simulink subsystem "WP_Guidance"  (R2021b)
settings: Solver=VariableStepAuto  StartTime=0.0  StopTime=10.0  RelTol=1e-3
undefined symbols (not defined in the file): ap, Earth, WGS84
libraries: mbdriLib x8, aerolibtransform2 x2
settings Model: Creator=promero  LastModifiedBy=promero

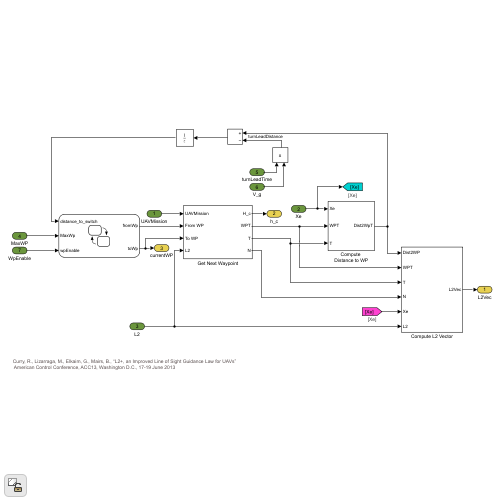
[thumbnail: Simulink's stored preview of the top-level diagram]
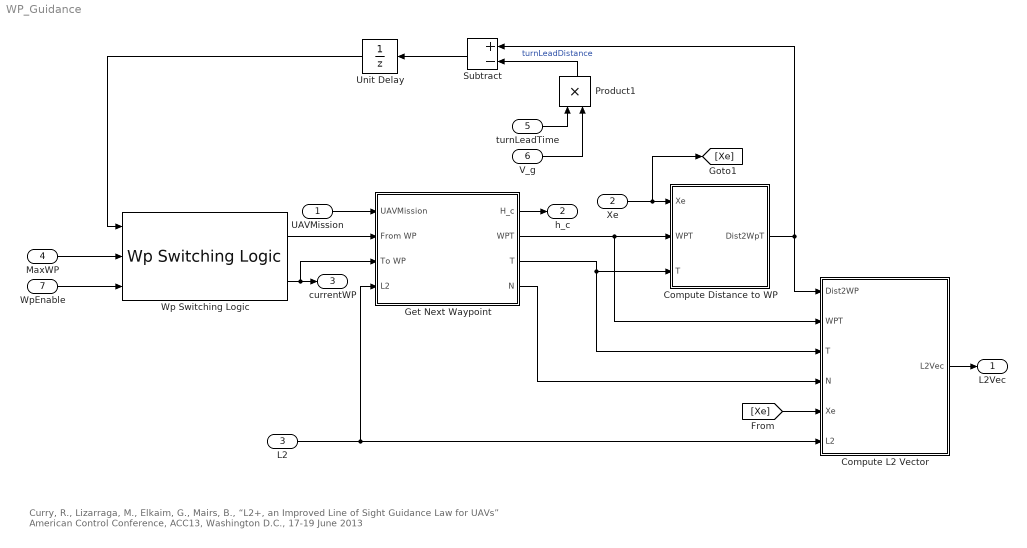
== system WP_Guidance ==
  note: Curry, R., Lizarraga, M., Elkaim, G., Mairs, B., “L2+, an Improved Line of Sight Guidance Law for UAVs”
      | American Control Conference, ACC13, Washington D.C., 17-19 June 2013
  UAVMission : Inport  RequirementInfo={} %GIDa_ee9cd0ca_ee46_4171_b2ca_c1436fe27e01
  Xe : Inport  RequirementInfo={} %GIDa_72129976_cf07_4668_8a2e_61079a25596c  Port=2
  L2 : Inport  RequirementInfo={} %GIDa_3bb9d2b1_49b6_4fd1_b19e_adcb7eb29e87  Port=3
  MaxWP : Inport  RequirementInfo={} %GIDa_a09e5540_0b09_46ae_86e8_d118108091d8  Port=4
  turnLeadTime : Inport  RequirementInfo={} %GIDa_310f2894_0be5_46e2_9beb_aa289b5e1983  Port=5
  V_g : Inport  RequirementInfo={} %GIDa_5e669477_500d_4a22_8597_17cbcbc01fd5  Port=6
  WpEnable : Inport  RequirementInfo={} %GIDa_1e5c6837_24ed_43c1_b836_520ffefd3b33  Port=7
  Compute Distance to WP : Subsystem  RequirementInfo={'linktype_rmi_slreq' 'electricUAVReqs.slreqx' '72' 'true' 'WP_GDNC_4: Distance To Waypoint Computation (electricUAVReqs#72)' '' } %GIDa_1a937859_3a63_446f_9abf_868d2299e4e6
  Compute L2 Vector : Subsystem  RequirementInfo={} %GIDa_5a423c49_5421_4da8_9f38_705098db439f
  Get Next Waypoint : Subsystem  RequirementInfo={} %GIDa_f2c23518_208d_4e4a_b1c3_dd5023478aa5
  Product1 : Product  RequirementInfo={'linktype_rmi_slreq' 'electricUAVReqs.slreqx' '73' 'true' 'WP_GDNC_5: Turn Lead Time on Waypoint Transition (electricUAVReqs#73)' '' } %GIDa_8680b81e_d9d6_452c_b3f7_0e38b456a447  OutDataTypeStr=single  RndMeth=Zero
  Subtract : Sum  RequirementInfo={'linktype_rmi_slreq' 'electricUAVReqs.slreqx' '73' 'true' 'WP_GDNC_5: Turn Lead Time on Waypoint Transition (electricUAVReqs#73)' '' } %GIDa_5f93a301_56af_4524_94ca_23c573592b7f  Inputs=+-
  Unit Delay : UnitDelay  RequirementInfo={} %GIDa_36c83432_323e_4005_b34d_2bf25e211813  InitialCondition=1000  SampleTime=-1  HasFrameUpgradeWarning=on
  Wp Switching Logic : mbdriLib/Guidance/Wp Switching Logic  SystemSampleTime=-1  VariantActivationTime=update diagram  Latency=0  AutoFrameSizeCalculation=off
  L2Vec : Outport  RequirementInfo={} %GIDa_92dd828a_6e6c_41ad_baca_94d61fc6dba3  VectorParamsAs1DForOutWhenUnconnected=off
  h_c : Outport  RequirementInfo={} %GIDa_750bd64b_af27_4708_ac3c_f4df04315bbb  Port=2  VectorParamsAs1DForOutWhenUnconnected=off
  currentWP : Outport  RequirementInfo={} %GIDa_3fd56a91_03a5_4a81_b62f_7152539b9a4e  Port=3  VectorParamsAs1DForOutWhenUnconnected=off
  wires:
  Get Next Waypoint/1(H_c) -> h_c/1
  [Xe] -> Compute L2 Vector/5(Xe)
  Wp Switching Logic/2 -> Get Next Waypoint/3(To WP), currentWP/1
  Get Next Waypoint/2(WPT) -> Compute Distance to WP/2(WPT), Compute L2 Vector/2(WPT)
  Compute Distance to WP/1(Dist2WpT) -> Compute L2 Vector/1(Dist2WP), Subtract/1
  Get Next Waypoint/3(T) -> Compute Distance to WP/3(T), Compute L2 Vector/3(T)
  Wp Switching Logic/1 -> Get Next Waypoint/2(From WP)
  V_g/1 -> Product1/2
  MaxWP/1 -> Wp Switching Logic/2
  L2/1 -> Compute L2 Vector/6(L2), Get Next Waypoint/4(L2)
  Get Next Waypoint/4(N) -> Compute L2 Vector/4(N)
  UAVMission/1 -> Get Next Waypoint/1(UAVMission)
  Compute L2 Vector/1(L2Vec) -> L2Vec/1
  Product1/1 -> Subtract/2  "turnLeadDistance"
  Subtract/1 -> Unit Delay/1
  turnLeadTime/1 -> Product1/1
  Unit Delay/1 -> Wp Switching Logic/1
  WpEnable/1 -> Wp Switching Logic/3
  Xe/1 -> Compute Distance to WP/1(Xe), [Xe]

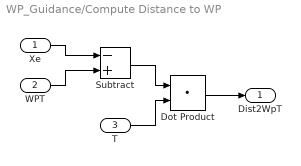
== system WP_Guidance/Compute Distance to WP ==
  Xe : Inport  RequirementInfo={} %GIDa_9f8d8236_2429_4b7b_a482_38fa48ab7648
  WPT : Inport  RequirementInfo={} %GIDa_d526967a_6982_4d7a_82b3_8316dae40b56  Port=2
  T : Inport  RequirementInfo={} %GIDa_11cd8214_427d_4f93_9bed_6a4eba75fbec  Port=3
  Dot Product : DotProduct  RequirementInfo={} %GIDa_e1a992b3_2ed6_4964_adf7_a3f8c3e62025  InputSameDT=on  OutDataTypeStr=Inherit: Inherit via internal rule
  Subtract : Sum  RequirementInfo={} %GIDa_3cfaf367_c734_4865_8f8b_705eb8be25de  Inputs=-+
  Dist2WpT : Outport  RequirementInfo={} %GIDa_f2f7793d_335a_403b_b52f_89e13dd8fb40  VectorParamsAs1DForOutWhenUnconnected=off
  wires:
  Dot Product/1 -> Dist2WpT/1
  Xe/1 -> Subtract/1
  WPT/1 -> Subtract/2
  Subtract/1 -> Dot Product/1
  T/1 -> Dot Product/2

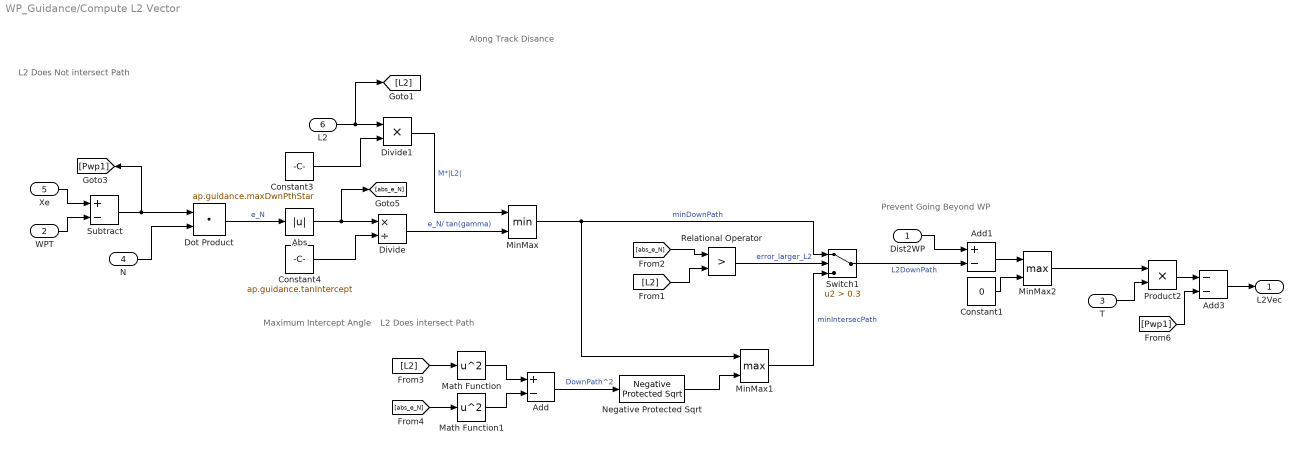
== system WP_Guidance/Compute L2 Vector ==
  note: Maximum Intercept Angle
  note: Along Track Disance
  note: L2 Does Not intersect Path
  note: L2 Does intersect Path
  note: Prevent Going Beyond WP
  Dist2WP : Inport  RequirementInfo={} %GIDa_e65bee0d_7cb0_4830_891e_2195d1cdaece
  WPT : Inport  RequirementInfo={} %GIDa_0976f7fa_1c01_43bb_ada1_9bdcc9a4c861  Port=2
  T : Inport  RequirementInfo={} %GIDa_ab04084b_cc55_4226_90a5_125cf357690c  Port=3
  N : Inport  RequirementInfo={} %GIDa_5029cf6e_d2cf_4233_9907_34e102b1998a  Port=4
  Xe : Inport  RequirementInfo={} %GIDa_7eca166f_3c2c_4a65_bba4_49777c34acaf  Port=5
  L2 : Inport  RequirementInfo={} %GIDa_6291a963_4b5b_4cef_8856_aece13d2d9a0  Port=6
  Abs : Abs  RequirementInfo={} %GIDa_98e47695_d57c_449a_bc4c_fc5551f2939e
  Add : Sum  RequirementInfo={} %GIDa_5fbdfcde_ce46_408f_a55b_ab1175565832  Inputs=+-
  Add1 : Sum  RequirementInfo={} %GIDa_5a227cf9_e434_444b_a630_b52d2e33683d  Inputs=+-
  Add3 : Sum  RequirementInfo={} %GIDa_05e4da75_772f_435f_aa92_8860f7b64972  Inputs=--
  Constant1 : Constant  RequirementInfo={} %GIDa_4615b8b3_bb6a_47fe_902a_54255cb7424f  Value=0
      settings: AttributesFormatString=%<Value>
  Constant3 : Constant  RequirementInfo={} %GIDa_0cfd4662_c184_4392_9461_495ddd94c08a  Value=ap.guidance.maxDwnPthStar
      settings: AttributesFormatString=%<Value>
  Constant4 : Constant  RequirementInfo={} %GIDa_d5fe3970_8fcf_4298_806a_062ef252a685  Value=ap.guidance.tanIntercept
      settings: AttributesFormatString=%<Value>
  Divide : Product  RequirementInfo={} %GIDa_935db90c_7b50_4f71_8b3b_176f49ab2bef  Inputs=*/
  Divide1 : Product  RequirementInfo={} %GIDa_1d972cff_4e14_44d2_8441_cc46c3cb282c
  Dot Product : DotProduct  RequirementInfo={} %GIDa_28268062_c71b_4a6e_96fb_eb131810d0a0  InputSameDT=on  OutDataTypeStr=Inherit: Inherit via internal rule
  Math Function : Math  RequirementInfo={} %GIDa_dbfe976e_428a_4583_8997_79c04f4bee07  Operator=square  SignedPower=on  SaturateOnIntegerOverflow=on
  Math Function1 : Math  RequirementInfo={} %GIDa_97787944_cd2b_4813_867f_005f37936185  Operator=square  SignedPower=on  SaturateOnIntegerOverflow=on
  MinMax : MinMax  RequirementInfo={'linktype_rmi_slreq' 'electricUAVReqs.slreqx' '81' 'true' 'WP_GDNC_10: Selecting a Minimum Path Distance for WP Guidance (electricUAVReqs#81)' '' } %GIDa_5c94b7a0_c9cb_45ac_8f52_ce17d08f50c9  Inputs=2
  MinMax1 : MinMax  RequirementInfo={'linktype_rmi_slreq' 'electricUAVReqs.slreqx' '82' 'true' 'WP_GDNC_10_1: Selecting L2 Down Path Distance (electricUAVReqs#82)' '' } %GIDa_9aa71b0d_c2a7_4613_b336_1e7a1ce45b38  Function=max  Inputs=2
  MinMax2 : MinMax  RequirementInfo={'linktype_rmi_slreq' 'electricUAVReqs.slreqx' '83' 'true' 'WP_GDNC_10_2: Avoiding Flying Beyond To Waypoint (electricUAVReqs#83)' '' } %GIDa_6e7a28a4_f0e0_4723_91cc_d00474509057  Function=max  Inputs=2
  Negative Protected Sqrt : mbdriLib/Utilities/Negative Protected Sqrt  RequirementInfo={} %GIDa_3d7354fd_42b9_4582_a03b_da800f1c5d08  SystemSampleTime=-1  VariantActivationTime=update diagram  Latency=0  AutoFrameSizeCalculation=off
  Product2 : Product  RequirementInfo={} %GIDa_23c8ccfd_b0bc_47eb_a4a9_10c64dd31921  RndMeth=Zero
  Relational Operator : RelationalOperator  RequirementInfo={} %GIDa_c5b23d8f_bfb5_4061_ac0b_fefb8a9677ff  Operator=>  OutDataTypeStr=boolean  RndMeth=Nearest
  Subtract : Sum  RequirementInfo={} %GIDa_06aceb5c_5a7e_4288_b3a6_acec342c55a0  Inputs=+-
  Switch1 : Switch  RequirementInfo={} %GIDa_13f7c6ad_1857_4e56_b3f0_e7e8676d7d2b  Criteria=u2 > Threshold  Threshold=0.3
  L2Vec : Outport  RequirementInfo={} %GIDa_89fe650a_dcb6_44d4_a1bf_5eac83b83fd8  VectorParamsAs1DForOutWhenUnconnected=off
  wires:
  Dist2WP/1 -> Add1/1
  N/1 -> Dot Product/2
  Add3/1 -> L2Vec/1
  [Pwp1] -> Add3/2
  Product2/1 -> Add3/1
  T/1 -> Product2/2
  MinMax2/1 -> Product2/1
  Constant1/1 -> MinMax2/2
  Add1/1 -> MinMax2/1
  MinMax1/1 -> Switch1/3  "minIntersecPath"
  Math Function1/1 -> Add/2
  [abs_e_N] -> Math Function1/1
  Math Function/1 -> Add/1
  [L2] -> Math Function/1
  Negative Protected Sqrt/1 -> MinMax1/2
  Add/1 -> Negative Protected Sqrt/1  "DownPath^2"
  Switch1/1 -> Add1/2  "L2DownPath"
  [abs_e_N] -> Relational Operator/1
  [L2] -> Relational Operator/2
  Relational Operator/1 -> Switch1/2  "error_larger_L2"
  MinMax/1 -> Switch1/1, MinMax1/1  "minDownPath"
  Divide1/1 -> MinMax/1  "M*|L2|"
  Constant3/1 -> Divide1/2
  L2/1 -> [L2], Divide1/1
  Divide/1 -> MinMax/2  "e_N/ tan(gamma)"
  Constant4/1 -> Divide/2
  Abs/1 -> [abs_e_N], Divide/1
  Dot Product/1 -> Abs/1  "e_N"
  Subtract/1 -> [Pwp1], Dot Product/1
  WPT/1 -> Subtract/2
  Xe/1 -> Subtract/1

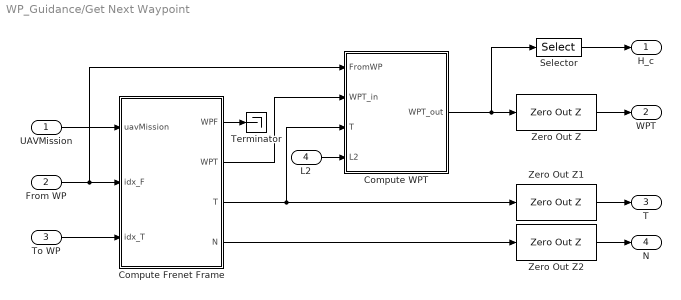
== system WP_Guidance/Get Next Waypoint ==
  UAVMission : Inport  RequirementInfo={} %GIDa_62966f62_afea_467c_b8c6_c495333b0227
  From WP : Inport  RequirementInfo={} %GIDa_60ab3fe3_46a4_4f0e_a9db_518a31a3c271  Port=2
  To WP : Inport  RequirementInfo={} %GIDa_f20a6783_74c1_46e7_a5b1_ba0de2aaadf5  Port=3
  L2 : Inport  RequirementInfo={} %GIDa_9fba8317_1c9f_4473_aab2_4b2c4ba25eb2  Port=4
  Compute Frenet Frame : Subsystem  RequirementInfo={} %GIDa_9942693d_5f68_4f68_bb34_4b0d87c140ce
  Compute WPT : Subsystem  RequirementInfo={} %GIDa_af75e753_7ce8_4a90_ae67_3227ab1538a8  TreatAsAtomicUnit=on
  Selector : Selector  RequirementInfo={} %GIDa_f465fccc_010d_4d99_98f4_e73f64c0afb9  InputPortWidth=3  IndexOptions=Index vector (dialog)  Indices=[3]  OutputSizes=1
  Terminator : Terminator
      settings: RequirementInfo={} %GIDa_7722b810_e5f1_4510_91fc_fa27a438450e
  Zero Out Z : mbdriLib/Utilities/Zero Out Z  RequirementInfo={} %GIDa_a4986d41_f410_4a06_926d_6769f51dfe4d  SystemSampleTime=-1  VariantActivationTime=update diagram  Latency=0  AutoFrameSizeCalculation=off
  Zero Out Z1 : mbdriLib/Utilities/Zero Out Z  RequirementInfo={} %GIDa_5b313be8_5a41_4419_92fe_210785bec891  SystemSampleTime=-1  VariantActivationTime=update diagram  Latency=0  AutoFrameSizeCalculation=off
  Zero Out Z2 : mbdriLib/Utilities/Zero Out Z  RequirementInfo={} %GIDa_64137d09_cb30_445e_85d7_73ce0c331a25  SystemSampleTime=-1  VariantActivationTime=update diagram  Latency=0  AutoFrameSizeCalculation=off
  H_c : Outport  RequirementInfo={} %GIDa_6f4309e1_4d4b_461d_8f6b_b4a36ad4ceec  VectorParamsAs1DForOutWhenUnconnected=off
  WPT : Outport  RequirementInfo={} %GIDa_0e85b784_cc11_42b3_a961_7b7906b051d7  Port=2  VectorParamsAs1DForOutWhenUnconnected=off
  T : Outport  RequirementInfo={} %GIDa_e74aa77e_ee40_4c29_8797_ff667a915573  Port=3  VectorParamsAs1DForOutWhenUnconnected=off
  N : Outport  RequirementInfo={} %GIDa_2c33e664_1cb0_4250_a371_feb0211cad7f  Port=4  VectorParamsAs1DForOutWhenUnconnected=off
  wires:
  Selector/1 -> H_c/1
  Zero Out Z/1 -> WPT/1
  L2/1 -> Compute WPT/4(L2)
  Compute Frenet Frame/2(WPT) -> Compute WPT/2(WPT_in)
  Compute WPT/1(WPT_out) -> Zero Out Z/1, Selector/1
  UAVMission/1 -> Compute Frenet Frame/1(uavMission)
  Zero Out Z2/1 -> N/1
  Zero Out Z1/1 -> T/1
  Compute Frenet Frame/4(N) -> Zero Out Z2/1
  Compute Frenet Frame/3(T) -> Zero Out Z1/1, Compute WPT/3(T)
  To WP/1 -> Compute Frenet Frame/3(idx_T)
  From WP/1 -> Compute Frenet Frame/2(idx_F), Compute WPT/1(FromWP)
  Compute Frenet Frame/1(WPF) -> Terminator/1

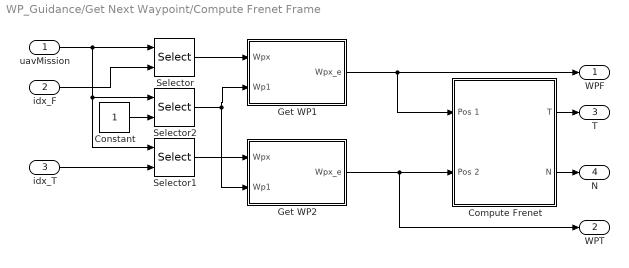
== system WP_Guidance/Get Next Waypoint/Compute Frenet Frame ==
  uavMission : Inport  RequirementInfo={} %GIDa_d3cfdd57_4ab9_418a_9c74_8cdd96f604ca
  idx_F : Inport  RequirementInfo={} %GIDa_de58cb5c_2287_4096_a9fc_36c54a43bc3a  Port=2
  idx_T : Inport  RequirementInfo={} %GIDa_180ae63a_faa8_4a13_8257_caa65714a956  Port=3
  Compute Frenet : Subsystem  RequirementInfo={'linktype_rmi_slreq' 'electricUAVReqs.slreqx' '74' 'true' 'WP_GDNC_6: Frenet Frame Computation (electricUAVReqs#74)' '' } %GIDa_4ffe5682_18da_43f5_b2a3_08dd7574ece1
  Constant : Constant  RequirementInfo={} %GIDa_5efc1e68_52e1_4b03_a568_739d35bb3b5d
      settings: AttributesFormatString=%<Value>
  Get WP1 : Subsystem  RequirementInfo={} %GIDa_41baa632_40d5_4e66_bbc0_01e1e7ace62c
  Get WP2 : Subsystem  RequirementInfo={} %GIDa_f6a96d7e_52bd_4233_9639_87ab2be25a8d
  Selector : Selector  RequirementInfo={} %GIDa_fc27a87a_5d46_45b9_9312_a8ff993dc8c4  InputPortWidth=10  IndexOptions=Index vector (port)  Indices=[1 3]  OutputSizes=1
  Selector1 : Selector  RequirementInfo={} %GIDa_709288d0_fa18_4477_b5b5_680492e73bce  InputPortWidth=10  IndexOptions=Index vector (port)  Indices=[1 3]  OutputSizes=1
  Selector2 : Selector  RequirementInfo={} %GIDa_cbc45855_550d_479f_b55f_3375b66b5dd0  InputPortWidth=10  IndexOptions=Index vector (port)  Indices=[1 3]  OutputSizes=1
  WPF : Outport  RequirementInfo={} %GIDa_9d2476bd_8fb9_46cb_916a_dfbaac0105c0  VectorParamsAs1DForOutWhenUnconnected=off
  WPT : Outport  RequirementInfo={} %GIDa_4bcbb536_3d7e_4627_81cb_b3182094e05a  Port=2  VectorParamsAs1DForOutWhenUnconnected=off
  T : Outport  RequirementInfo={} %GIDa_5cc83c8c_f0c2_463b_a682_667b8d903cad  Port=3  VectorParamsAs1DForOutWhenUnconnected=off
  N : Outport  RequirementInfo={} %GIDa_ea044ad4_3bdb_4c9f_8842_bc17fad46e89  Port=4  VectorParamsAs1DForOutWhenUnconnected=off
  wires:
  Selector2/1 -> Get WP2/2(Wp1), Get WP1/2(Wp1)
  Constant/1 -> Selector2/2
  idx_T/1 -> Selector1/2
  idx_F/1 -> Selector/2
  Get WP1/1(Wpx_e) -> WPF/1, Compute Frenet/1(Pos 1)
  Selector1/1 -> Get WP2/1(Wpx)
  Selector/1 -> Get WP1/1(Wpx)
  uavMission/1 -> Selector/1, Selector1/1, Selector2/1
  Compute Frenet/1(T) -> T/1
  Compute Frenet/2(N) -> N/1
  Get WP2/1(Wpx_e) -> Compute Frenet/2(Pos 2), WPT/1

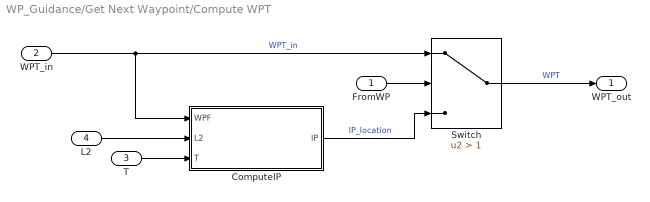
== system WP_Guidance/Get Next Waypoint/Compute WPT ==
  FromWP : Inport  RequirementInfo={} %GIDa_c5b173f4_7825_4972_84b2_574c42726ff5
  WPT_in : Inport  RequirementInfo={} %GIDa_f92e1e36_ba2c_419f_9473_a1526fc797ee  Port=2
  T : Inport  RequirementInfo={} %GIDa_0b30cbcc_d4f5_44cc_bcf6_b39f19d23cc6  Port=3
  L2 : Inport  RequirementInfo={} %GIDa_f8191a58_4627_40ba_9cfc_516877fe1e99  Port=4
  ComputeIP : Subsystem  RequirementInfo={'linktype_rmi_slreq' 'electricUAVReqs.slreqx' '75' 'true' 'WP_GDNC_7: Initial Point Computation (electricUAVReqs#75)' '' } %GIDa_4240619b_f424_4970_98d1_275fd1fd5306
  Switch : Switch  RequirementInfo={'linktype_rmi_slreq' 'electricUAVReqs.slreqx' '80' 'true' 'WP_GDNC_2_2: WPT Computation when in TO_IP State (electricUAVReqs#80)' '' ; 'linktype_rmi_slreq' 'electricUAVReqs.slreqx' '78' 'true' 'WP_GDNC_9: To Waypoint Calculation (electricUAVReqs#78)' '' } %GIDa_f0e653d3_2824_433d_a731_343bedbf0159  Criteria=u2 > Threshold  Threshold=1
  WPT_out : Outport  RequirementInfo={} %GIDa_512da935_36b7_4cef_8d10_1e545ec1afb3  VectorParamsAs1DForOutWhenUnconnected=off
  wires:
  WPT_in/1 -> ComputeIP/1(WPF), Switch/1  "WPT_in"
  FromWP/1 -> Switch/2
  Switch/1 -> WPT_out/1  "WPT"
  L2/1 -> ComputeIP/2(L2)
  T/1 -> ComputeIP/3(T)
  ComputeIP/1(IP) -> Switch/3  "IP_location"

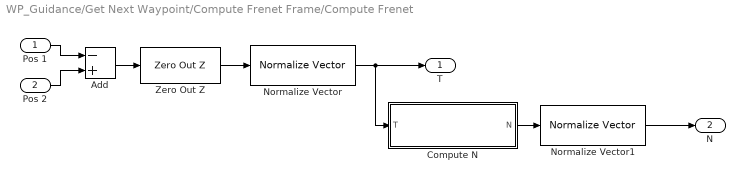
== system WP_Guidance/Get Next Waypoint/Compute Frenet Frame/Compute Frenet ==
  Pos 1 : Inport  RequirementInfo={} %GIDa_68cf308f_211d_4fdf_aa59_416ba1bce983
  Pos 2 : Inport  RequirementInfo={} %GIDa_941529b7_ab98_41c8_ad89_f48eedcb0596  Port=2
  Add : Sum  RequirementInfo={} %GIDa_be6bac2a_c1e9_476d_a9a5_6621eba6144d  Inputs=-+
  Compute N : Subsystem  RequirementInfo={} %GIDa_1b84684b_3574_4a2a_b0d6_f0ad4e63eb85
  Normalize Vector : mbdriLib/Utilities/Normalize Vector  RequirementInfo={} %GIDa_ad48d3dd_6035_46e8_b816_67ba6393bcf1  SystemSampleTime=-1  VariantActivationTime=update diagram  Latency=0  AutoFrameSizeCalculation=off
  Normalize Vector1 : mbdriLib/Utilities/Normalize Vector  RequirementInfo={} %GIDa_0184db18_27a4_4ca7_8e4d_0f78ba1957e8  SystemSampleTime=-1  VariantActivationTime=update diagram  Latency=0  AutoFrameSizeCalculation=off
  Zero Out Z : mbdriLib/Utilities/Zero Out Z  RequirementInfo={} %GIDa_cad817f2_6b8e_4272_b32d_53c4bf1ae935  SystemSampleTime=-1  VariantActivationTime=update diagram  Latency=0  AutoFrameSizeCalculation=off
  T : Outport  RequirementInfo={} %GIDa_94942750_a589_4af6_8be8_1db32435de33  VectorParamsAs1DForOutWhenUnconnected=off
  N : Outport  RequirementInfo={} %GIDa_580b8fb7_8836_4b14_ac97_c112fbed111f  Port=2  VectorParamsAs1DForOutWhenUnconnected=off
  wires:
  Compute N/1(N) -> Normalize Vector1/1
  Pos 1/1 -> Add/1
  Pos 2/1 -> Add/2
  Add/1 -> Zero Out Z/1
  Normalize Vector1/1 -> N/1
  Normalize Vector/1 -> Compute N/1(T), T/1
  Zero Out Z/1 -> Normalize Vector/1

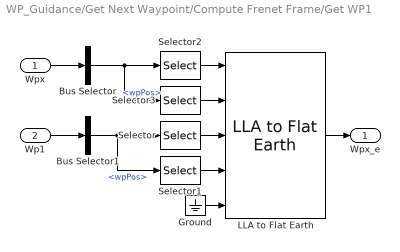
== system WP_Guidance/Get Next Waypoint/Compute Frenet Frame/Get WP1 ==
  Wpx : Inport  RequirementInfo={} %GIDa_06ae3dd0_5af6_4cba_be39_3b3f7ceb21d1  OutDataTypeStr=Bus: waypoint
  Wp1 : Inport  RequirementInfo={} %GIDa_5839b076_c279_4ccf_87d7_0b27a76e3303  Port=2  OutDataTypeStr=Bus: waypoint
  Bus Selector : BusSelector  RequirementInfo={} %GIDa_aff3978a_760d_43ac_9a6d_6a946b8d7341  OutputSignals=wpPos
  Bus Selector1 : BusSelector  RequirementInfo={} %GIDa_f19bf213_5c3e_40d1_b872_9fac5bd2e0df  OutputSignals=wpPos
  Ground : Ground  RequirementInfo={} %GIDa_f1919ed9_1f84_49dd_afb1_bae91276483e
  LLA to Flat Earth : aerolibtransform2/LLA to Flat Earth  RequirementInfo={} %GIDa_a2d73b17_4238_48ed_9f5b_af67c64a7ea9  units=Metric (MKS)  ptype=Earth (WGS84)  F=1/298.257223563  R=6378137  refPosPort=on  LL0=[0 10]  psi=0
      settings: SourceProductBaseCode=AE
  Selector : Selector  RequirementInfo={} %GIDa_b17f2f05_e28f_4e33_8ba3_d40e871f2bd9  InputPortWidth=3  IndexOptions=Index vector (dialog)  Indices=[3]  OutputSizes=1
  Selector1 : Selector  RequirementInfo={} %GIDa_515ff3cb_26f1_4fa6_ac00_1bb6c98ace76  InputPortWidth=3  IndexOptions=Index vector (dialog)  Indices=[1 2]  OutputSizes=1
  Selector2 : Selector  RequirementInfo={} %GIDa_63a27cef_91d8_4eb5_b7cf_c5ee591aa256  InputPortWidth=3  IndexOptions=Index vector (dialog)  Indices=[1 2]  OutputSizes=1
  Selector3 : Selector  RequirementInfo={} %GIDa_6b4fb6bc_2f61_40c0_8ec3_c37d2fd71cd6  InputPortWidth=3  IndexOptions=Index vector (dialog)  Indices=[3]  OutputSizes=1
  Wpx_e : Outport  RequirementInfo={} %GIDa_43061348_f790_4bd2_917f_b7e41465b1d3  VectorParamsAs1DForOutWhenUnconnected=off
  wires:
  Selector3/1 -> LLA to Flat Earth/2
  Selector2/1 -> LLA to Flat Earth/1
  Bus Selector1/1 -> Selector/1, Selector1/1  "<wpPos>"
  Wp1/1 -> Bus Selector1/1
  Bus Selector/1 -> Selector2/1, Selector3/1  "<wpPos>"
  Wpx/1 -> Bus Selector/1
  Selector1/1 -> LLA to Flat Earth/4
  Selector/1 -> LLA to Flat Earth/3
  LLA to Flat Earth/1 -> Wpx_e/1
  Ground/1 -> LLA to Flat Earth/5

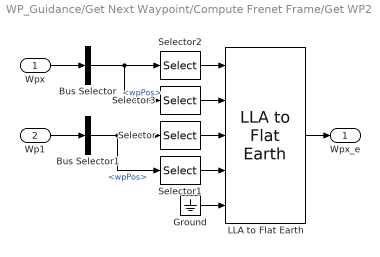
== system WP_Guidance/Get Next Waypoint/Compute Frenet Frame/Get WP2 ==
  Wpx : Inport  RequirementInfo={} %GIDa_3c81a71c_dd6b_4404_9bab_d08fb36c7b30  OutDataTypeStr=Bus: waypoint
  Wp1 : Inport  RequirementInfo={} %GIDa_544d1763_e334_493c_899c_f8b6966ea4b4  Port=2  OutDataTypeStr=Bus: waypoint
  Bus Selector : BusSelector  RequirementInfo={} %GIDa_680a472c_d9b9_4a23_b56a_60766d44bc47  OutputSignals=wpPos
  Bus Selector1 : BusSelector  RequirementInfo={} %GIDa_9985f2e3_362f_47b5_8f73_1981d8e1b414  OutputSignals=wpPos
  Ground : Ground  RequirementInfo={} %GIDa_2aa30dd1_b5b8_4cc6_8a67_c49e9cdefb1e
  LLA to Flat Earth : aerolibtransform2/LLA to Flat Earth  RequirementInfo={} %GIDa_35a4d861_bd52_473b_bf41_20c097df65b5  units=Metric (MKS)  ptype=Earth (WGS84)  F=1/298.257223563  R=6378137  refPosPort=on  LL0=[0 10]  psi=0
      settings: SourceProductBaseCode=AE
  Selector : Selector  RequirementInfo={} %GIDa_5f09b62d_9e71_4cf3_b191_2c823fc0a5fc  InputPortWidth=3  IndexOptions=Index vector (dialog)  Indices=[3]  OutputSizes=1
  Selector1 : Selector  RequirementInfo={} %GIDa_fc05efd3_08d9_46e3_a43e_8c786f4ed09e  InputPortWidth=3  IndexOptions=Index vector (dialog)  Indices=[1 2]  OutputSizes=1
  Selector2 : Selector  RequirementInfo={} %GIDa_78a1da67_34f5_48ec_8e59_b2040042f6a6  InputPortWidth=3  IndexOptions=Index vector (dialog)  Indices=[1 2]  OutputSizes=1
  Selector3 : Selector  RequirementInfo={} %GIDa_65ee098a_8982_40e8_8afd_cdd5d19ba697  InputPortWidth=3  IndexOptions=Index vector (dialog)  Indices=[3]  OutputSizes=1
  Wpx_e : Outport  RequirementInfo={} %GIDa_213b9b8f_42f5_4803_a1c7_694cbaf764ad  VectorParamsAs1DForOutWhenUnconnected=off
  wires:
  LLA to Flat Earth/1 -> Wpx_e/1
  Selector/1 -> LLA to Flat Earth/3
  Selector1/1 -> LLA to Flat Earth/4
  Wpx/1 -> Bus Selector/1
  Bus Selector/1 -> Selector3/1, Selector2/1  "<wpPos>"
  Wp1/1 -> Bus Selector1/1
  Bus Selector1/1 -> Selector1/1, Selector/1  "<wpPos>"
  Selector2/1 -> LLA to Flat Earth/1
  Selector3/1 -> LLA to Flat Earth/2
  Ground/1 -> LLA to Flat Earth/5

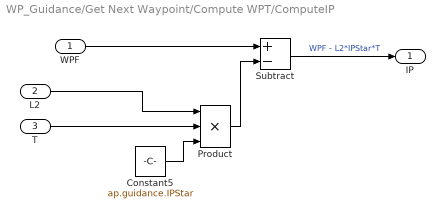
== system WP_Guidance/Get Next Waypoint/Compute WPT/ComputeIP ==
  WPF : Inport  RequirementInfo={} %GIDa_5443ed4c_b1e0_4370_bc77_af127f7bdbb0
  L2 : Inport  RequirementInfo={} %GIDa_edf28ade_e910_4b59_a1db_1dc5391d7f11  Port=2
  T : Inport  RequirementInfo={} %GIDa_a345a127_342d_40e4_94a6_8c0bc0ca9b44  Port=3
  Constant5 : Constant  RequirementInfo={} %GIDa_4ab98dba_8d16_4e31_a942_87a7857b8baa  Value=ap.guidance.IPStar
      settings: AttributesFormatString=%<Value>
  Product : Product  RequirementInfo={} %GIDa_a0329e8b_2d35_4bbe_8e10_1797daca7c4a  Inputs=3  RndMeth=Zero
  Subtract : Sum  RequirementInfo={} %GIDa_c0ccd6ba_27b7_4335_a1c7_d0e945b5b21b  Inputs=+-
  IP : Outport  RequirementInfo={} %GIDa_14a408bc_3d23_4521_951b_91e20a8d46a5  VectorParamsAs1DForOutWhenUnconnected=off
  wires:
  Subtract/1 -> IP/1  "WPF - L2*IPStar*T"
  T/1 -> Product/2
  L2/1 -> Product/1
  WPF/1 -> Subtract/1
  Product/1 -> Subtract/2
  Constant5/1 -> Product/3

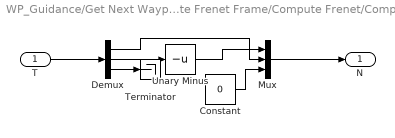
== system WP_Guidance/Get Next Waypoint/Compute Frenet Frame/Compute Frenet/Compute N ==
  T : Inport  RequirementInfo={} %GIDa_02e835e3_ef1f_4c25_8d21_db0098590ed6
  Constant : Constant  RequirementInfo={} %GIDa_0f0cff7f_89cb_4ed0_9f8b_7e142b336d36  Value=0
      settings: AttributesFormatString=%<Value>
  Demux : Demux  RequirementInfo={} %GIDa_3b9e8acb_f05f_48fa_b43d_3ca22cacfdfd  Outputs=3
  Mux : Mux  RequirementInfo={} %GIDa_00239762_7af6_47e3_8be3_64602d97bef0  Inputs=3
  Terminator : Terminator
      settings: RequirementInfo={} %GIDa_090c697f_7db1_4ac0_a0d1_fc2600dee04c
  Unary Minus : UnaryMinus  RequirementInfo={} %GIDa_0e8f03cf_1a64_46af_b8c6_73aa57396aca
  N : Outport  RequirementInfo={} %GIDa_148f9f3c_7dcd_4a5b_b5d1_175062b6c074  VectorParamsAs1DForOutWhenUnconnected=off
  wires:
  Mux/1 -> N/1
  T/1 -> Demux/1
  Demux/1 -> Mux/2
  Constant/1 -> Mux/3
  Demux/2 -> Unary Minus/1
  Unary Minus/1 -> Mux/1
  Demux/3 -> Terminator/1
